simulink model "SystemDynamics"  (R2024b)
settings: Solver=FixedStepAuto  StartTime=0.0  StopTime=5  FixedStep=0.001  RelTol=1e-3
values from neighbouring files (symbols this model uses):
  K = lqr(A_num,B_num,Q,R)    [solution.m]
  theta0 = pi-0.1    (= 3.04159265359)    [main.m]
  thetadot0 = 0    [main.m]
  Vin = 0    [main.m]    (also in pendulum_dynamics.m = max(min(Vin,24),-24))
  x0 = 0    [main.m]
  xdot0 = 0    [main.m]
undefined symbols (not defined in the file or in its folder): params
settings Model: Creator=samir  LastModifiedBy=samir
settings SolverCC: MaxConsecutiveMinStep=10
settings DebuggingCC: SignalInfNanChecking=error

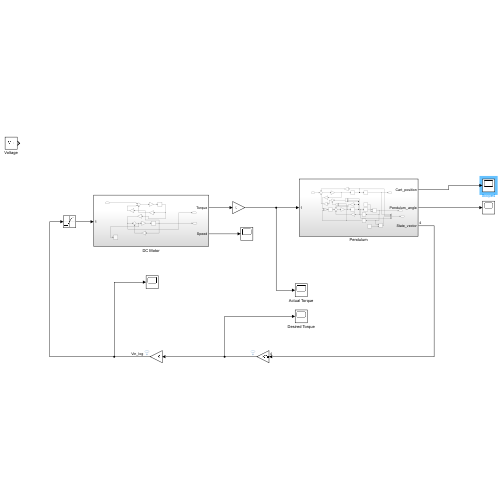
[thumbnail: Simulink's stored preview of the top-level diagram]
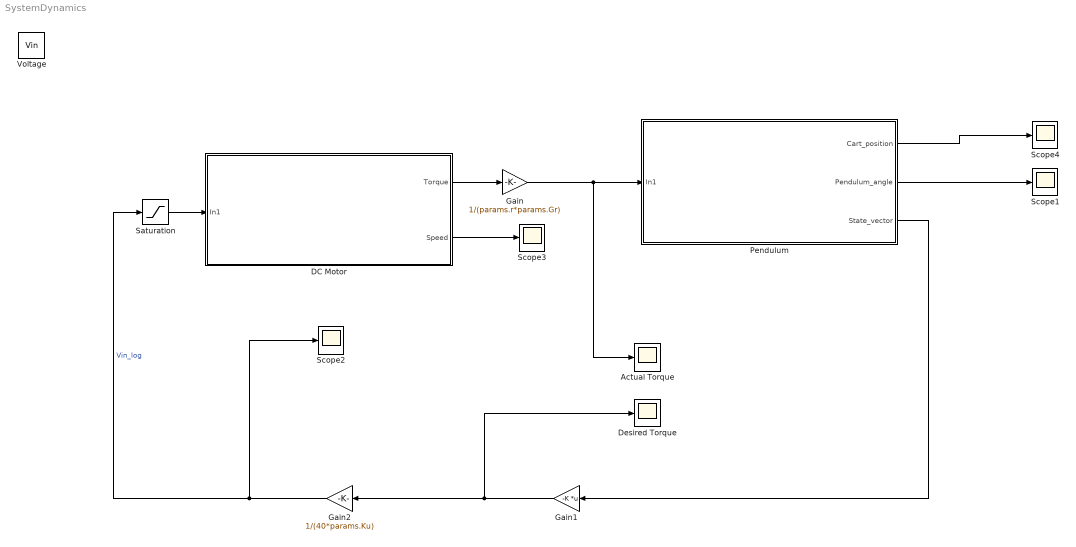
== system SystemDynamics ==
  Actual Torque : Scope
  DC Motor : Subsystem
  Desired Torque : Scope
  Gain : Gain  Gain=1/(params.r*params.Gr)
  Gain1 : Gain  Gain=-K  Multiplication=Matrix(K*u)
  Gain2 : Gain  Gain=1/(40*params.Ku)
  Pendulum : Subsystem
  Saturation : Saturate  UpperLimit=24  LowerLimit=-24
  Scope{1..4} (4 alike) : Scope
  Voltage : Constant  Value=Vin
  wires:
  DC Motor/1(Torque) -> Gain/1
  Pendulum/3(State_vector) -> Gain1/1
  Gain1/1 -> Gain2/1, Desired Torque/1
  Pendulum/2(Pendulum_angle) -> Scope1/1
  Gain2/1 -> Scope2/1, Saturation/1  "Vin_log"
  DC Motor/2(Speed) -> Scope3/1
  Saturation/1 -> DC Motor/1(In1)
  Gain/1 -> Actual Torque/1, Pendulum/1(In1)
  Pendulum/1(Cart_position) -> Scope4/1

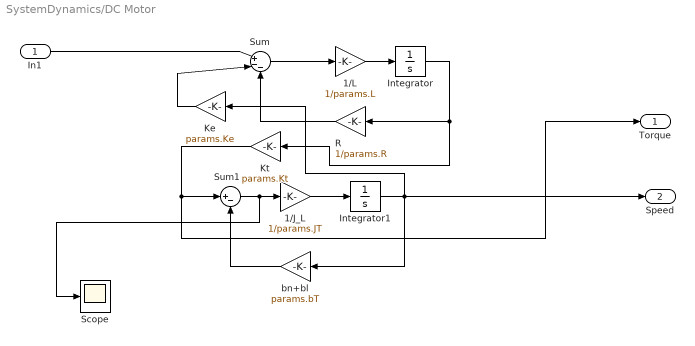
== system SystemDynamics/DC Motor ==
  In1 : Inport
  1/J_L : Gain  Gain=1/params.JT
  1/L : Gain  Gain=1/params.L
  Integrator : Integrator
  Integrator1 : Integrator
  Ke : Gain  Gain=params.Ke
  Kt : Gain  Gain=params.Kt
  R : Gain  Gain=1/params.R
  Scope : Scope
  Sum : Sum  Inputs=|+--
  Sum1 : Sum  Inputs=|+-
  bn+bl : Gain  Gain=params.bT
  Torque : Outport
  Speed : Outport  Port=2
  wires:
  Sum1/1 -> 1/J_L/1, Scope/1
  Ke/1 -> Sum/2
  Sum/1 -> 1/L/1
  Integrator1/1 -> bn+bl/1, Speed/1, Ke/1
  Kt/1 -> Sum1/1, Torque/1
  Integrator/1 -> Kt/1, R/1
  1/L/1 -> Integrator/1
  R/1 -> Sum/3
  bn+bl/1 -> Sum1/2
  In1/1 -> Sum/1
  1/J_L/1 -> Integrator1/1

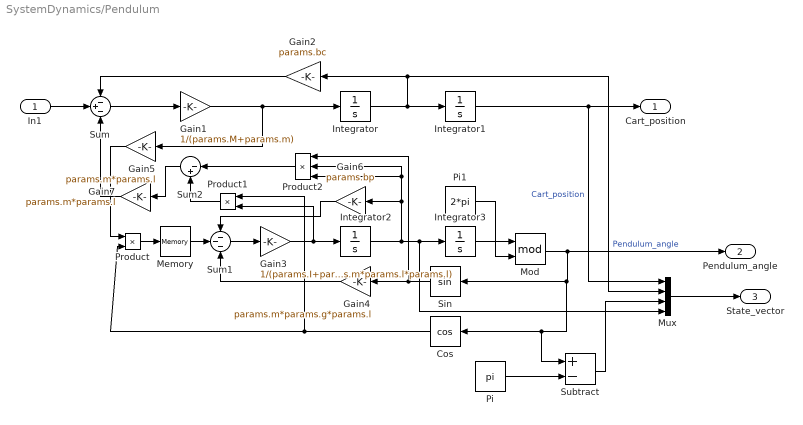
== system SystemDynamics/Pendulum ==
  In1 : Inport
  Cos : Trigonometry  Operator=cos
  Gain1 : Gain  Gain=1/(params.M+params.m)
  Gain2 : Gain  Gain=params.bc
  Gain3 : Gain  Gain=1/(params.I+params.m*params.l*params.l)
  Gain4 : Gain  Gain=params.m*params.g*params.l
  Gain5 : Gain  Gain=params.m*params.l
  Gain6 : Gain  Gain=params.bp
  Gain7 : Gain  Gain=params.m*params.l
  Integrator : Integrator  InitialCondition=xdot0
  Integrator1 : Integrator  InitialCondition=x0
  Integrator2 : Integrator  InitialCondition=thetadot0
  Integrator3 : Integrator  InitialCondition=theta0
  Memory : Memory
  Mod : Math  Operator=mod
  Mux : Mux
  Pi : Constant  Value=pi  OutDataTypeStr=Inherit: Inherit via back propagation
  Pi1 : Constant  Value=2*pi  OutDataTypeStr=Inherit: Inherit via back propagation
  Product : Product
  Product1 : Product
  Product2 : Product  Inputs=3
  Sin : Trigonometry
  Subtract : Sum  Inputs=+-
  Sum : Sum  Inputs=-+-
  Sum1 : Sum  Inputs=---
  Sum2 : Sum  Inputs=|-+
  Cart_position : Outport
  Pendulum_angle : Outport  Port=2
  State_vector : Outport  Port=3
  wires:
  Sin/1 -> Product2/1, Gain4/1
  Integrator/1 -> Integrator1/1, Mux/2, Gain2/1
  Integrator3/1 -> Mod/1
  Gain1/1 -> Integrator/1, Gain5/1
  Cos/1 -> Product1/1, Product/2
  Sum/1 -> Gain1/1
  Gain7/1 -> Sum/3
  Integrator2/1 -> Mux/4, Integrator3/1, Gain6/1, Product2/2, Product2/3
  Sum2/1 -> Gain7/1
  Sum1/1 -> Gain3/1
  Product/1 -> Memory/1
  Gain3/1 -> Product1/2, Integrator2/1
  Gain4/1 -> Sum1/3
  Gain6/1 -> Sum1/1
  Product2/1 -> Sum2/1
  In1/1 -> Sum/2
  Gain2/1 -> Sum/1
  Product1/1 -> Sum2/2
  Gain5/1 -> Product/1
  Integrator1/1 -> Mux/1, Cart_position/1  "Cart_position"
  Memory/1 -> Sum1/2
  Mux/1 -> State_vector/1
  Pi/1 -> Subtract/2
  Subtract/1 -> Mux/3
  Pi1/1 -> Mod/2
  Mod/1 -> Subtract/1, Cos/1, Sin/1, Pendulum_angle/1  "Pendulum_angle"
